simulink model "System_discrete"  (R2020a)
settings: Solver=FixedStepAuto  StartTime=0.0  StopTime=10  RelTol=1e-3
undefined symbols (not defined in the file or in its folder): Ao, Bd, Bo, DiscIntNeverNeededParam, K_lqi_pc, Ki_d, La, sys_d, Te
libraries: simulink x1
settings Model: Creator=antoi  LastModifiedBy=antoi
settings SolverCC: AutoInsertRateTranBlk=on
settings OptimizationCC: DefaultParameterBehavior=Inlined  UseDivisionForNetSlopeComputation=on  GainParamInheritBuiltInType=on  UseFloatMulNetSlope=on  OptimizeBlockIOStorage=off  PassReuseOutputArgsThreshold=0  OptimizeDataStoreBuffers=off  BusAssignmentInplaceUpdate=off
settings DebuggingCC: ParameterTunabilityLossMsg=error  SFUnexpectedBacktrackingDiag=warning  SFNoUnconditionalDefaultTransitionDiag=warning
settings HardwareCC: ProdLongLongMode=on
settings SFSimCC: MATLABDynamicMemAlloc=off
settings RTWCC: Description=Generic Real-Time Target  GenerateReport=on  BuildConfiguration=Debug  LaunchReport=on
settings CodeAppCC: ForceParamTrailComments=on  OperatorAnnotations=on  MATLABSourceComments=on  EnableCustomComments=on
settings GRTTargetCC: CombineSignalStateStructs=on  SupportVariableSizeSignals=on  MultiInstanceErrorCode=Warning

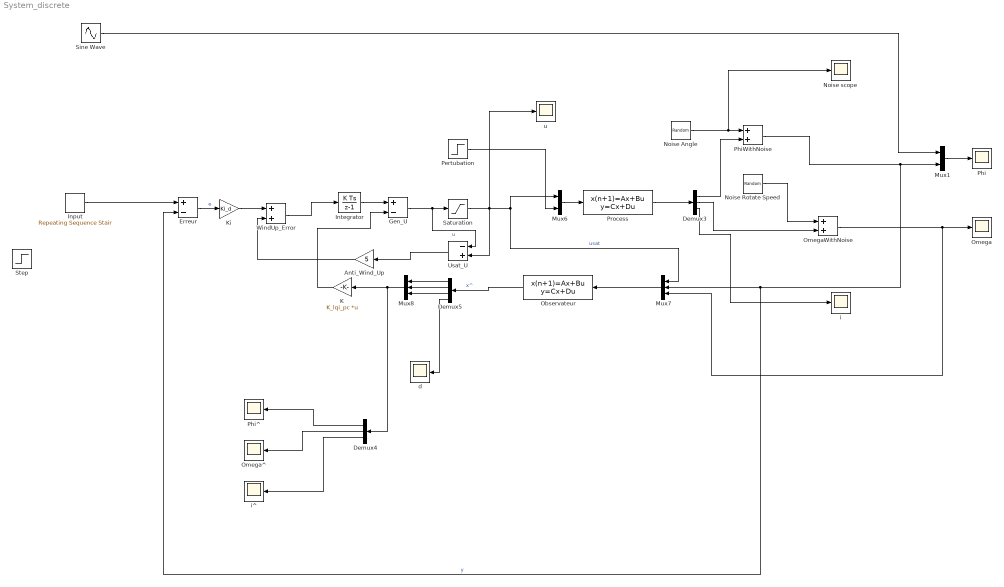
== system System_discrete ==
  Anti_Wind_Up : Gain  Gain=5
  Demux3 : Demux  Outputs=3
  Demux4 : Demux  Outputs=3
  Demux5 : Demux
  Erreur : Sum  Inputs=+-
  Gen_U : Sum  Inputs=+-
  Input : simulink/Sources/Repeating Sequence Stair  OutValues=[1 -1]'  tsamp=0.5  OutMin=[]  OutMax=[]  OutDataTypeStr=double  OutputDataTypeScalingMode=double  OutDataType=fixdt(0,8)  ConRadixGroup=Best Precision: Vector-wise  OutScaling=2^-12
  Integrator : DiscreteIntegrator  SampleTime=Te  ICPrevOutput=DiscIntNeverNeededParam  ICPrevScaledInput=DiscIntNeverNeededParam
  K : Gain  Gain=K_lqi_pc  Multiplication=Matrix(K*u) (u vector)
  Ki : Gain  Gain=Ki_d
  Mux1 : Mux  Inputs=2
  Mux6 : Mux  Inputs=2
  Mux7 : Mux  Inputs=3
  Mux8 : Mux  Inputs=3
  "Noise Angle " : RandomNumber  Variance=0  SampleTime=0.1
  Noise Rotate Speed : RandomNumber  Variance=0  SampleTime=0.1
  Noise scope : Scope
  Observateur : DiscreteStateSpace  A=Ao - La*[1 1 0 0]  B=[Bo La La]  C=eye(4)  D=[0 0 0; 0 0 0 ;0 0 0;0 0 0]  SampleTime=Te
  Omega : Scope
  OmegaWithNoise : Sum
  Omega^ : Scope
  Pertubation : Step  Time=3  After=0  SampleTime=0
  Phi : Scope
  PhiWithNoise : Sum
  Phi^ : Scope
  Process : DiscreteStateSpace  A=sys_d.a  B=[sys_d.b Bd]  C=eye(3)  D=[0 0; 0 0; 0 0]  SampleTime=Te
  Saturation : Saturate  UpperLimit=12  LowerLimit=-12
  Sine Wave : Sin  Frequency=6.2831853  Phase=pi  SampleTime=0
  Step : Step  SampleTime=0
  Usat_U : Sum  Inputs=-+
  WindUp_Error : Sum
  d : Scope
  i : Scope
  i^ : Scope
  u : Scope
  wires:
  Usat_U/1 -> Anti_Wind_Up/1
  Demux5/3 -> Mux8/3
  Mux1/1 -> Phi/1
  Anti_Wind_Up/1 -> WindUp_Error/2
  Gen_U/1 -> Usat_U/1, Saturation/1  "u"
  Demux5/2 -> Mux8/2
  OmegaWithNoise/1 -> Mux7/3, Omega/1
  Demux5/1 -> Mux8/1
  WindUp_Error/1 -> Integrator/1
  Mux8/1 -> Demux4/1, K/1
  Pertubation/1 -> Mux6/2
  Noise Rotate Speed/1 -> OmegaWithNoise/1
  Demux3/2 -> OmegaWithNoise/2
  Saturation/1 -> Usat_U/2, Mux6/1, Mux7/1, u/1  "usat"
  Erreur/1 -> Ki/1  "e"
  Ki/1 -> WindUp_Error/1
  Demux4/3 -> i^/1
  Demux3/1 -> PhiWithNoise/2
  Demux3/3 -> i/1
  Demux4/2 -> Omega^/1
  Demux5/4 -> d/1
  K/1 -> Gen_U/2
  Demux4/1 -> Phi^/1
  Integrator/1 -> Gen_U/1
  Mux6/1 -> Process/1
  Process/1 -> Demux3/1
  Mux7/1 -> Observateur/1
  Observateur/1 -> Demux5/1  "x^"
  "Noise Angle "/1 -> PhiWithNoise/1, Noise scope/1
  PhiWithNoise/1 -> Mux7/2, Erreur/2, Mux1/2  "y"
  Input/1 -> Erreur/1
  Sine Wave/1 -> Mux1/1
